simulink model "Electric_System"  (R2016b)
settings: Solver=FixedStepDiscrete  StartTime=0.0  StopTime=inf  FixedStep=ElecSys.tiSimnTiStep_C.Value  RelTol=1e-3  EnableMultiTasking=on
settings Model: Creator=djuenema  LastModifiedBy=djuenema
settings DataIOCC: SaveFormat=StructureWithTime  SaveOutput=off  DSMLogging=off  VisualizeSimOutput=off  SaveTime=off  SignalLoggingName=Results
settings OptimizationCC: BlockReduction=off  ConditionallyExecuteInputs=off  LifeSpan=inf
settings DebuggingCC: AllowSymbolicDim=off  SFUnexpectedBacktrackingDiag=warning  SFNoUnconditionalDefaultTransitionDiag=warning  SFExecutionAtInitializationDiag=none
settings ModelReferenceCC: ModelReferenceNumInstancesAllowed=Single  PropagateSignalLabelsOutOfModel=off
settings GRTTargetCC: TargetLangStandard=C89/C90 (ANSI)
settings ConfigComp: CovMetricSettings=dw  CovHtmlReporting=on  CovSaveCumulativeToWorkspaceVar=on  CovSaveSingleToWorkspaceVar=on  CovExternalEMLEnable=off

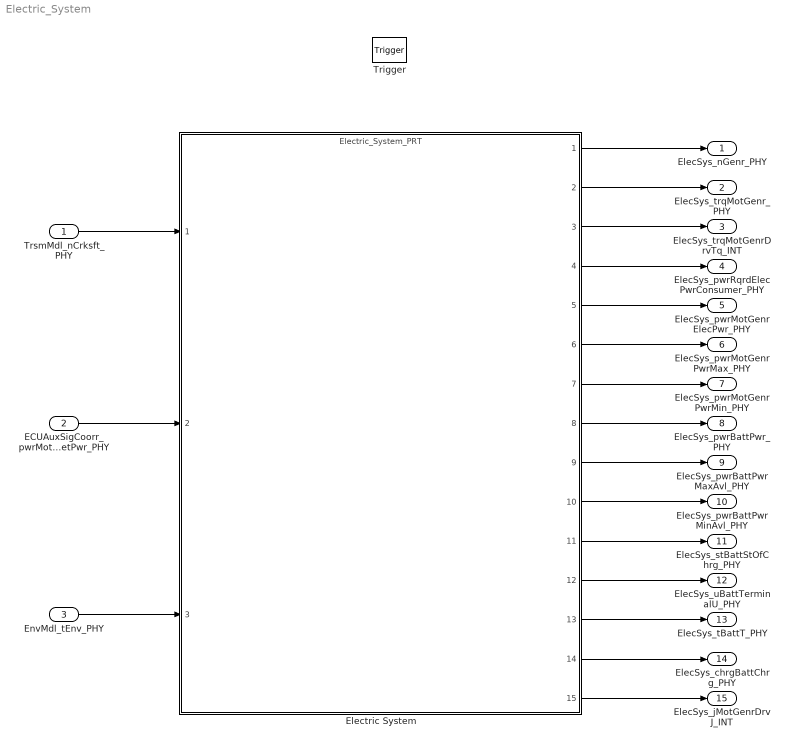
== system Electric_System ==
  TrsmMdl_nCrksft_PHY : Inport
  ECUAuxSigCoorr_pwrMotGenrSetPwr_PHY : Inport  Port=2
  EnvMdl_tEnv_PHY : Inport  Port=3
  Trigger : TriggerPort  TriggerType=function-call  VariantControl=Variant  PortDimensions=1
  Electric System : ModelReference  ModelNameDialog=Electric_System_PRT.slxp  ModelReferenceVersion=1.3  CopyOfModelProtected=on
  ElecSys_nGenr_PHY : Outport
  ElecSys_trqMotGenr_PHY : Outport  Port=2
  ElecSys_trqMotGenrDrvTq_INT : Outport  Port=3
  ElecSys_pwrRqrdElecPwrConsumer_PHY : Outport  Port=4
  ElecSys_pwrMotGenrElecPwr_PHY : Outport  Port=5
  ElecSys_pwrMotGenrPwrMax_PHY : Outport  Port=6
  ElecSys_pwrMotGenrPwrMin_PHY : Outport  Port=7
  ElecSys_pwrBattPwr_PHY : Outport  Port=8
  ElecSys_pwrBattPwrMaxAvl_PHY : Outport  Port=9
  ElecSys_pwrBattPwrMinAvl_PHY : Outport  Port=10
  ElecSys_stBattStOfChrg_PHY : Outport  Port=11
  ElecSys_uBattTerminalU_PHY : Outport  Port=12
  ElecSys_tBattT_PHY : Outport  Port=13
  ElecSys_chrgBattChrg_PHY : Outport  Port=14
  ElecSys_jMotGenrDrvJ_INT : Outport  Port=15
  wires:
  TrsmMdl_nCrksft_PHY/1 -> Electric System/1
  ECUAuxSigCoorr_pwrMotGenrSetPwr_PHY/1 -> Electric System/2
  EnvMdl_tEnv_PHY/1 -> Electric System/3
  Electric System/1 -> ElecSys_nGenr_PHY/1
  Electric System/2 -> ElecSys_trqMotGenr_PHY/1
  Electric System/4 -> ElecSys_pwrRqrdElecPwrConsumer_PHY/1
  Electric System/3 -> ElecSys_trqMotGenrDrvTq_INT/1
  Electric System/5 -> ElecSys_pwrMotGenrElecPwr_PHY/1
  Electric System/15 -> ElecSys_jMotGenrDrvJ_INT/1
  Electric System/6 -> ElecSys_pwrMotGenrPwrMax_PHY/1
  Electric System/7 -> ElecSys_pwrMotGenrPwrMin_PHY/1
  Electric System/8 -> ElecSys_pwrBattPwr_PHY/1
  Electric System/9 -> ElecSys_pwrBattPwrMaxAvl_PHY/1
  Electric System/10 -> ElecSys_pwrBattPwrMinAvl_PHY/1
  Electric System/11 -> ElecSys_stBattStOfChrg_PHY/1
  Electric System/12 -> ElecSys_uBattTerminalU_PHY/1
  Electric System/13 -> ElecSys_tBattT_PHY/1
  Electric System/14 -> ElecSys_chrgBattChrg_PHY/1
